simulink model "gm_DUALportRAMinterface_v3_vnl"  (R2024a)
settings: Solver=FixedStepDiscrete  StartTime=0.0  StopTime=0.1  RelTol=1e-3
undefined symbols (not defined in the file or in its folder): magnitude, Ts
libraries: hdlsllib x227, embmathops x6, simulink x2, hdlmdlgenlib x1, dsphdlxfrm2 x1
(part 1 of 6)
settings Model: Creator=Simon  LastModifiedBy=Simon
settings OptimizationCC: BlockReduction=off  ConditionallyExecuteInputs=off  DefaultParameterBehavior=Inlined  InheritOutputTypeSmallerThanSingle=on
settings DebuggingCC: AlgebraicLoopMsg=error  InheritedTsInSrcMsg=none  SingleTaskRateTransMsg=error  UnconnectedInputMsg=warning  UnconnectedOutputMsg=warning  UnconnectedLineMsg=warning
settings HardwareCC: ProdBitPerPointer=32  ProdBitPerSizeT=32  ProdBitPerPtrDiffT=32  ProdLargestAtomicFloat=None  ProdIntDivRoundTo=Undefined  ProdEndianess=Unspecified  ProdWordSize=32  ProdHWDeviceType=ASIC/FPGA->ASIC/FPGA  TargetBitPerPointer=64  TargetBitPerSizeT=64  TargetBitPerPtrDiffT=64  TargetLongLongMode=on  TargetIntDivRoundTo=Zero  TargetEndianess=LittleEndian  TargetWordSize=64  TargetHWDeviceType=Custom Processor->MATLAB Host Computer  ProdEqTarget=off

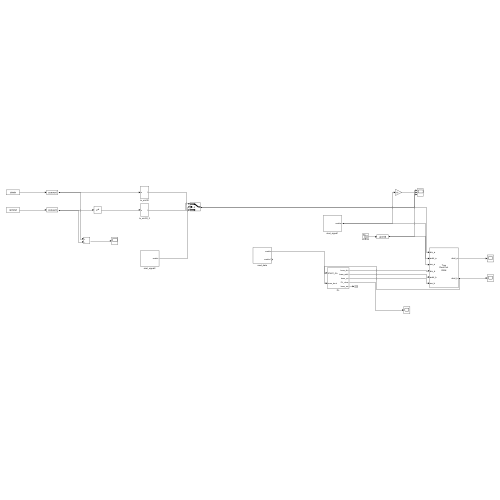
[thumbnail: Simulink's stored preview of the top-level diagram]
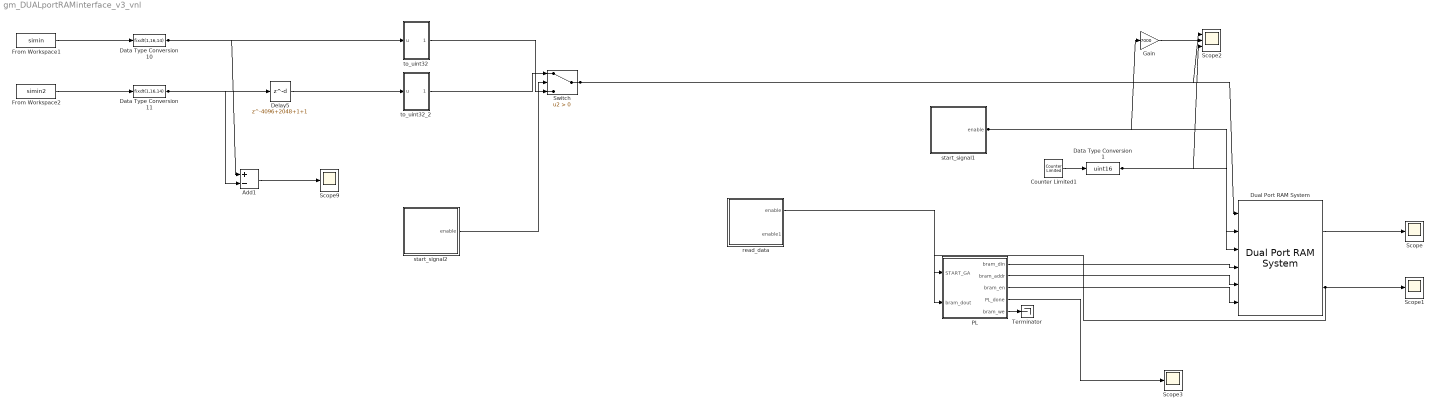
== system gm_DUALportRAMinterface_v3_vnl ==
  Add1 : Sum  Inputs=+-
  Counter Limited1 : simulink/Sources/Counter Limited  uplimit=14000  tsamp=Ts
  Data Type Conversion1 : DataTypeConversion  OutDataTypeStr=uint16  SaturateOnIntegerOverflow=off  RndMeth=Floor
  Data Type Conversion10 : DataTypeConversion  OutDataTypeStr=fixdt(1,16,14)  SaturateOnIntegerOverflow=off  RndMeth=Floor
  Data Type Conversion11 : DataTypeConversion  OutDataTypeStr=fixdt(1,16,14)  SaturateOnIntegerOverflow=off  RndMeth=Floor
  Delay5 : Delay  DelayLength=4096+2048+1+1  InitialCondition=0  SampleTime=Ts
  Dual Port RAM System : hdlsllib/HDL RAMs/Dual Port RAM System  RAMType=True dual port  AsyncRead=off  WriteOutputValue=New data  RAMInitialValue=0  allowBusInputs=off  WritesHaveOutput=on  NumReads=0  NumWrites=1  SimulateUsing=Code generation
  From Workspace1 : FromWorkspace  VariableName=simin  SampleTime=Ts
  From Workspace2 : FromWorkspace  VariableName=simin2  SampleTime=Ts
  Gain : Gain  Gain=7000
  PL : Subsystem
  Scope{,1,3,9} (4 alike) : Scope
  Scope2 : Scope  NumInputPorts=3
  Switch : Switch  Criteria=u2 > Threshold  SaturateOnIntegerOverflow=off  InputSameDT=off  OutDataTypeStr=Inherit: Same as first input
  Terminator : Terminator
  read_data : Subsystem
  start_signal1 : Subsystem
  start_signal2 : Subsystem
  to_uint32 : Subsystem
  to_uint32_2 : Subsystem
  wires:
  PL/5(bram_we) -> Terminator/1
  PL/4(PL_done) -> Scope3/1
  Data Type Conversion10/1 -> to_uint32/1(u), Add1/1
  Add1/1 -> Scope9/1
  Data Type Conversion11/1 -> Add1/2, Delay5/1
  Switch/1 -> Dual Port RAM System/1, Scope2/1
  Delay5/1 -> to_uint32_2/1(u)
  start_signal2/1(enable) -> Switch/2
  to_uint32_2/1(Out1) -> Switch/1
  to_uint32/1(Out1) -> Switch/3
  From Workspace2/1 -> Data Type Conversion11/1
  From Workspace1/1 -> Data Type Conversion10/1
  Dual Port RAM System/2 -> PL/2(bram_dout), Scope1/1
  read_data/1(enable) -> PL/1(START_GA)
  Gain/1 -> Scope2/2
  PL/3(bram_en) -> Dual Port RAM System/6
  PL/2(bram_addr) -> Dual Port RAM System/5
  PL/1(bram_din) -> Dual Port RAM System/4
  start_signal1/1(enable) -> Gain/1, Dual Port RAM System/3
  Data Type Conversion1/1 -> Dual Port RAM System/2, Scope2/3
  Counter Limited1/1 -> Data Type Conversion1/1
  Dual Port RAM System/1 -> Scope/1

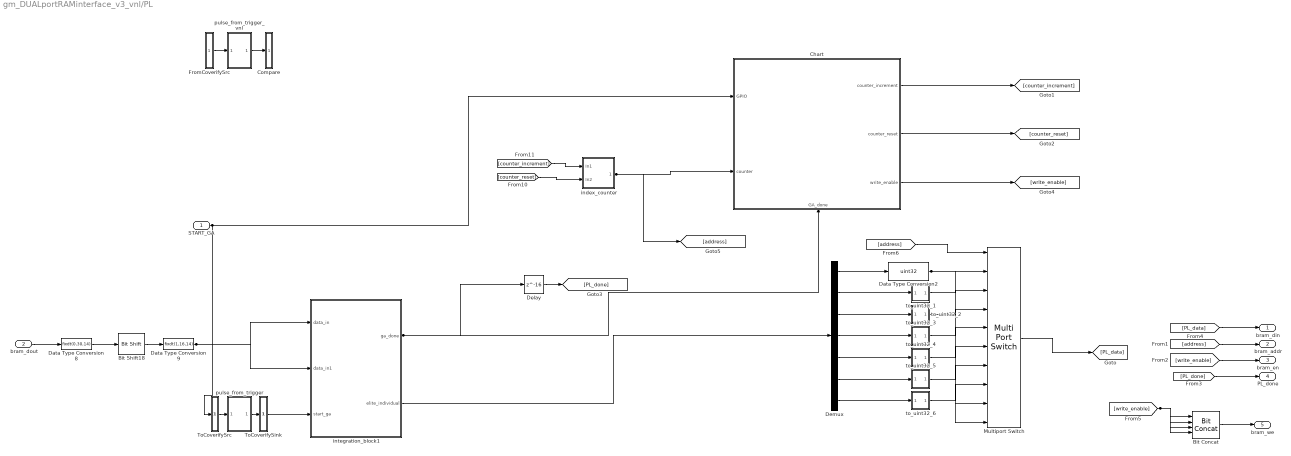
== system gm_DUALportRAMinterface_v3_vnl/PL ==
  START_GA : Inport
  bram_dout : Inport  Port=2
  Bit Concat : hdlsllib/Logic and Bit Operations/Bit Concat  numInputs=4
  Bit Shift18 : hdlsllib/Logic and Bit Operations/Bit Shift  mode=Shift Right Logical  N=14
  Chart : Stateflow chart  TreatAsAtomicUnit=on
      settings: PortSchema="{\"entries\":[{\"content\":{\"sides\":[{\"content\":{\"connectorIds\":[\"In2\",\"In3\"]},\"type\":\"ConnectorPlacement.EquallySpacedRectSide\",\"uuid\":\"f3ce331f-c708-4668-a9cb-fb327ea74ab5\"},{\"content\":{\"connectorIds\":[\"Out1\",\"Out2\",\"Out3\"],\"side\":\"RIGHT\"},\"type\":\"ConnectorPlacement.EquallySpacedRectSide\",\"uuid\":\"3766927a-abff-497d-9544-2098881ba174\"},{\"content\":{\"side\":\"TOP\"},\"type\":\"ConnectorPlacement.EquallySpacedRectSide\",\"uuid\":\"ebfe3d64-ee7d-4953-a6ba-e7e40988decf\"},{\"content\":{\"connectorIds\":[\"In1\"],\"side\":\"BOTTOM\"},\"type\":\"ConnectorPlacement.EquallySpacedRectSide\",\"uuid\":\"f39ceaf8-4df7-4e40-9de5-da7597831fb4\"}]},\"type\":\"ConnectorPlacement.EquallySpacedConnector\",\"uuid\":\"89f60450-5933-42bb-b72b-5f8ec55483e0\"}],\"packageUris\":[\"http://schema.mathworks.com/mf0/Connector/R2020b\"],\"version\":\"1.0\"}"
  Compare : Subsystem
      mask Display: disp('')
  Data Type Conversion2 : DataTypeConversion  OutDataTypeStr=uint32  SaturateOnIntegerOverflow=off  RndMeth=Floor
  Data Type Conversion8 : DataTypeConversion  OutDataTypeStr=fixdt(0,30,14)  SaturateOnIntegerOverflow=off  RndMeth=Floor
  Data Type Conversion9 : DataTypeConversion  OutDataTypeStr=fixdt(1,16,14)  SaturateOnIntegerOverflow=off  RndMeth=Floor
  Delay : Delay  DelayLength=16  InitialCondition=0  SampleTime=Ts
  Demux : Demux  Outputs=7
  FromCoverifySrc : Subsystem
      mask Display: disp('')
  Multiport Switch : MultiPortSwitch  DataPortOrder=Specify indices  Inputs=8  DataPortIndices={0,1,2,3,4,5,6,7}  DataPortForDefault=Additional data port  DiagnosticForDefault=None  SaturateOnIntegerOverflow=off  InputSameDT=off
  ToCoverifySink : Subsystem
      mask Display: disp('')
  ToCoverifySrc : Subsystem
      mask Display: disp('')
  index_counter : Subsystem
  integration_block1 : Subsystem
  pulse_from_trigger : Subsystem
  pulse_from_trigger_vnl : Subsystem
  to_uint32_1 : Subsystem
  to_uint32_2 : Subsystem
  to_uint32_3 : Subsystem
  to_uint32_4 : Subsystem
  to_uint32_5 : Subsystem
  to_uint32_6 : Subsystem
  bram_din : Outport
  bram_addr : Outport  Port=2
  bram_en : Outport  Port=3
  PL_done : Outport  Port=4
  bram_we : Outport  Port=5
  wires:
  Multiport Switch/1 -> [PL_data]
  [counter_reset] -> index_counter/2(In2)
  index_counter/1(index_counter) -> Chart/3(counter), [address]
  [address] -> bram_addr/1
  [counter_increment] -> index_counter/1(In1)
  [address] -> Multiport Switch/1
  Chart/3(write_enable) -> [write_enable]
  integration_block1/1(ga_done) -> Delay/1, Chart/1(GA_done)
  START_GA/1 -> Chart/2(GPIO), ToCoverifySrc/1(in1)
  Chart/2(counter_reset) -> [counter_reset]
  Chart/1(counter_increment) -> [counter_increment]
  [PL_data] -> bram_din/1
  [write_enable] -> bram_en/1
  integration_block1/2(elite_individual) -> Demux/1
  Demux/1 -> Data Type Conversion2/1
  Demux/2 -> to_uint32_1/1(u_port)
  Demux/3 -> to_uint32_2/1(u_port)
  Demux/4 -> to_uint32_3/1(u_port)
  Demux/5 -> to_uint32_4/1(u_port)
  Demux/6 -> to_uint32_5/1(u_port)
  Demux/7 -> to_uint32_6/1(u_port)
  Data Type Conversion2/1 -> Multiport Switch/10, Multiport Switch/9, Multiport Switch/2
  to_uint32_1/1(Out1) -> Multiport Switch/3
  to_uint32_2/1(Out1) -> Multiport Switch/4
  to_uint32_3/1(Out1) -> Multiport Switch/5
  to_uint32_4/1(Out1) -> Multiport Switch/6
  to_uint32_5/1(Out1) -> Multiport Switch/7
  to_uint32_6/1(Out1) -> Multiport Switch/8
  Data Type Conversion9/1 -> integration_block1/1(data_in), integration_block1/2(data_in1)
  Bit Shift18/1 -> Data Type Conversion9/1
  Data Type Conversion8/1 -> Bit Shift18/1
  bram_dout/1 -> Data Type Conversion8/1
  [PL_done] -> PL_done/1
  Delay/1 -> [PL_done]
  Bit Concat/1 -> bram_we/1
  [write_enable] -> Bit Concat/4, Bit Concat/3, Bit Concat/2, Bit Concat/1
  ToCoverifySrc/1(out1) -> pulse_from_trigger/1(In1)
  pulse_from_trigger/1(Out1) -> ToCoverifySink/1(in1)
  ToCoverifySink/1(out1) -> integration_block1/3(start_ga)
  FromCoverifySrc/1(out1) -> pulse_from_trigger_vnl/1(In1)
  pulse_from_trigger_vnl/1(Out1) -> Compare/1(in1)

== system gm_DUALportRAMinterface_v3_vnl/read_data ==
  Data Type Conversion1 : DataTypeConversion  Commented=on  OutDataTypeStr=boolean  SaturateOnIntegerOverflow=off  RndMeth=Floor
  Data Type Conversion29 : DataTypeConversion  OutDataTypeStr=boolean  SaturateOnIntegerOverflow=off  RndMeth=Floor
  Delay1 : Delay  Commented=on  DelayLength=1  InitialCondition=0  SampleTime=Ts
  Gain : Gain
  Gain1 : Gain  Commented=on
  Step1 : Step  Time=Ts*14000  SampleTime=Ts
  Step2 : Step  Commented=on  Time=Ts*14000  SampleTime=Ts
  XOR2 : Logic  Commented=on  Operator=XOR  IconShape=distinctive  AllPortsSameDT=off  OutDataTypeStr=boolean
  enable : Outport
  enable1 : Outport  Port=2
  wires:
  Gain1/1 -> Data Type Conversion1/1
  Step2/1 -> XOR2/1, Delay1/1
  Delay1/1 -> XOR2/2
  XOR2/1 -> Gain1/1
  Data Type Conversion1/1 -> enable1/1
  Data Type Conversion29/1 -> enable/1
  Gain/1 -> Data Type Conversion29/1
  Step1/1 -> Gain/1

== system gm_DUALportRAMinterface_v3_vnl/start_signal1 ==
  Data Type Conversion29 : DataTypeConversion  OutDataTypeStr=boolean  SaturateOnIntegerOverflow=off  RndMeth=Floor
  Delay2 : Delay  DelayLength=(4096+2048+1+1)*2  InitialCondition=0  SampleTime=Ts
  Gain : Gain
  Step1 : Step  Time=Ts*0  SampleTime=Ts
  XOR1 : Logic  Operator=XOR  IconShape=distinctive  AllPortsSameDT=off  OutDataTypeStr=boolean
  enable : Outport
  wires:
  XOR1/1 -> Gain/1
  Step1/1 -> Delay2/1, XOR1/1
  Delay2/1 -> XOR1/2
  Gain/1 -> Data Type Conversion29/1
  Data Type Conversion29/1 -> enable/1

== system gm_DUALportRAMinterface_v3_vnl/start_signal2 ==
  Data Type Conversion29 : DataTypeConversion  OutDataTypeStr=boolean  SaturateOnIntegerOverflow=off  RndMeth=Floor
  Delay2 : Delay  DelayLength=(4096+2048+1+1)*2  InitialCondition=0  SampleTime=Ts
  Gain : Gain
  Step1 : Step  Time=Ts*(4096+2048+1+1)  SampleTime=Ts
  XOR1 : Logic  Operator=XOR  IconShape=distinctive  AllPortsSameDT=off  OutDataTypeStr=boolean
  enable : Outport
  wires:
  Data Type Conversion29/1 -> enable/1
  Gain/1 -> Data Type Conversion29/1
  Delay2/1 -> XOR1/2
  Step1/1 -> XOR1/1, Delay2/1
  XOR1/1 -> Gain/1

== system gm_DUALportRAMinterface_v3_vnl/to_uint32 ==
  u : Inport
  Bit Concat2 : hdlsllib/Logic and Bit Operations/Bit Concat  numInputs=16
  Bit Shift19 : hdlsllib/Logic and Bit Operations/Bit Shift  mode=Shift Left Logical  N=1
  Bit Shift20 : hdlsllib/Logic and Bit Operations/Bit Shift  mode=Shift Left Logical  N=10
  Bit Shift21 : hdlsllib/Logic and Bit Operations/Bit Shift  mode=Shift Right Logical  N=1
  Bit Shift22 : hdlsllib/Logic and Bit Operations/Bit Shift  mode=Shift Left Logical  N=11
  Bit Shift23 : hdlsllib/Logic and Bit Operations/Bit Shift  mode=Shift Left Logical  N=12
  Bit Shift24 : hdlsllib/Logic and Bit Operations/Bit Shift  mode=Shift Left Logical  N=13
  Bit Shift25 : hdlsllib/Logic and Bit Operations/Bit Shift  mode=Shift Left Logical  N=14
  Bit Shift26 : hdlsllib/Logic and Bit Operations/Bit Shift  mode=Shift Left Logical  N=2
  Bit Shift27 : hdlsllib/Logic and Bit Operations/Bit Shift  mode=Shift Left Logical  N=3
  Bit Shift28 : hdlsllib/Logic and Bit Operations/Bit Shift  mode=Shift Left Logical  N=4
  Bit Shift29 : hdlsllib/Logic and Bit Operations/Bit Shift  mode=Shift Left Logical  N=5
  Bit Shift30 : hdlsllib/Logic and Bit Operations/Bit Shift  mode=Shift Left Logical  N=6
  Bit Shift31 : hdlsllib/Logic and Bit Operations/Bit Shift  mode=Shift Left Logical  N=7
  Bit Shift32 : hdlsllib/Logic and Bit Operations/Bit Shift  mode=Shift Left Logical  N=8
  Bit Shift33 : hdlsllib/Logic and Bit Operations/Bit Shift  mode=Shift Left Logical  N=9
  Data Type Conversion{12..16,26,34..43} (16 alike) : DataTypeConversion  OutDataTypeStr=fixdt(0,1,0)  SaturateOnIntegerOverflow=off  RndMeth=Floor
  Data Type Conversion44 : DataTypeConversion  OutDataTypeStr=uint32  SaturateOnIntegerOverflow=off  RndMeth=Floor
  Out1 : Outport
  wires:
  Data Type Conversion14/1 -> Bit Concat2/10
  Bit Concat2/1 -> Data Type Conversion44/1
  Bit Shift26/1 -> Data Type Conversion35/1
  Bit Shift21/1 -> Data Type Conversion13/1
  Bit Shift28/1 -> Data Type Conversion26/1
  Data Type Conversion37/1 -> Bit Concat2/16
  Bit Shift29/1 -> Data Type Conversion16/1
  Bit Shift23/1 -> Data Type Conversion39/1
  Data Type Conversion41/1 -> Bit Concat2/12
  Bit Shift24/1 -> Data Type Conversion38/1
  Bit Shift33/1 -> Data Type Conversion42/1
  Data Type Conversion16/1 -> Bit Concat2/7
  Data Type Conversion43/1 -> Bit Concat2/9
  Data Type Conversion34/1 -> Bit Concat2/5
  Data Type Conversion39/1 -> Bit Concat2/14
  Bit Shift32/1 -> Data Type Conversion14/1
  Data Type Conversion12/1 -> Bit Concat2/2
  Bit Shift30/1 -> Data Type Conversion15/1
  Data Type Conversion15/1 -> Bit Concat2/8
  Bit Shift25/1 -> Data Type Conversion37/1
  Data Type Conversion38/1 -> Bit Concat2/15
  Bit Shift19/1 -> Data Type Conversion36/1
  Data Type Conversion42/1 -> Bit Concat2/11
  Data Type Conversion35/1 -> Bit Concat2/4
  Data Type Conversion44/1 -> Out1/1
  Data Type Conversion26/1 -> Bit Concat2/6
  Bit Shift31/1 -> Data Type Conversion43/1
  Data Type Conversion40/1 -> Bit Concat2/13
  Data Type Conversion13/1 -> Bit Concat2/1
  Bit Shift20/1 -> Data Type Conversion41/1
  u/1 -> Bit Shift25/1, Bit Shift24/1, Bit Shift23/1, Bit Shift22/1, Bit Shift20/1, Bit Shift33/1, Bit Shift32/1, Bit Shift31/1, Bit Shift30/1, Bit Shift29/1, Bit Shift28/1, Bit Shift27/1, Bit Shift26/1, Bit Shift19/1, Data Type Conversion12/1, Bit Shift21/1
  Data Type Conversion36/1 -> Bit Concat2/3
  Bit Shift27/1 -> Data Type Conversion34/1
  Bit Shift22/1 -> Data Type Conversion40/1

== system gm_DUALportRAMinterface_v3_vnl/to_uint32_2 ==
  u : Inport
  Bit Concat2 : hdlsllib/Logic and Bit Operations/Bit Concat  numInputs=16
  Bit Shift19 : hdlsllib/Logic and Bit Operations/Bit Shift  mode=Shift Left Logical  N=1
  Bit Shift20 : hdlsllib/Logic and Bit Operations/Bit Shift  mode=Shift Left Logical  N=10
  Bit Shift21 : hdlsllib/Logic and Bit Operations/Bit Shift  mode=Shift Right Logical  N=1
  Bit Shift22 : hdlsllib/Logic and Bit Operations/Bit Shift  mode=Shift Left Logical  N=11
  Bit Shift23 : hdlsllib/Logic and Bit Operations/Bit Shift  mode=Shift Left Logical  N=12
  Bit Shift24 : hdlsllib/Logic and Bit Operations/Bit Shift  mode=Shift Left Logical  N=13
  Bit Shift25 : hdlsllib/Logic and Bit Operations/Bit Shift  mode=Shift Left Logical  N=14
  Bit Shift26 : hdlsllib/Logic and Bit Operations/Bit Shift  mode=Shift Left Logical  N=2
  Bit Shift27 : hdlsllib/Logic and Bit Operations/Bit Shift  mode=Shift Left Logical  N=3
  Bit Shift28 : hdlsllib/Logic and Bit Operations/Bit Shift  mode=Shift Left Logical  N=4
  Bit Shift29 : hdlsllib/Logic and Bit Operations/Bit Shift  mode=Shift Left Logical  N=5
  Bit Shift30 : hdlsllib/Logic and Bit Operations/Bit Shift  mode=Shift Left Logical  N=6
  Bit Shift31 : hdlsllib/Logic and Bit Operations/Bit Shift  mode=Shift Left Logical  N=7
  Bit Shift32 : hdlsllib/Logic and Bit Operations/Bit Shift  mode=Shift Left Logical  N=8
  Bit Shift33 : hdlsllib/Logic and Bit Operations/Bit Shift  mode=Shift Left Logical  N=9
  Data Type Conversion{12..16,26,34..43} (16 alike) : DataTypeConversion  OutDataTypeStr=fixdt(0,1,0)  SaturateOnIntegerOverflow=off  RndMeth=Floor
  Data Type Conversion44 : DataTypeConversion  OutDataTypeStr=uint32  SaturateOnIntegerOverflow=off  RndMeth=Floor
  Out1 : Outport
  wires:
  Bit Shift22/1 -> Data Type Conversion40/1
  Bit Shift27/1 -> Data Type Conversion34/1
  Data Type Conversion36/1 -> Bit Concat2/3
  u/1 -> Bit Shift21/1, Data Type Conversion12/1, Bit Shift19/1, Bit Shift26/1, Bit Shift27/1, Bit Shift28/1, Bit Shift29/1, Bit Shift30/1, Bit Shift31/1, Bit Shift32/1, Bit Shift33/1, Bit Shift20/1, Bit Shift22/1, Bit Shift23/1, Bit Shift24/1, Bit Shift25/1
  Bit Shift20/1 -> Data Type Conversion41/1
  Data Type Conversion13/1 -> Bit Concat2/1
  Data Type Conversion40/1 -> Bit Concat2/13
  Bit Shift31/1 -> Data Type Conversion43/1
  Data Type Conversion26/1 -> Bit Concat2/6
  Data Type Conversion44/1 -> Out1/1
  Data Type Conversion35/1 -> Bit Concat2/4
  Data Type Conversion42/1 -> Bit Concat2/11
  Bit Shift19/1 -> Data Type Conversion36/1
  Data Type Conversion38/1 -> Bit Concat2/15
  Bit Shift25/1 -> Data Type Conversion37/1
  Data Type Conversion15/1 -> Bit Concat2/8
  Bit Shift30/1 -> Data Type Conversion15/1
  Data Type Conversion12/1 -> Bit Concat2/2
  Bit Shift32/1 -> Data Type Conversion14/1
  Data Type Conversion39/1 -> Bit Concat2/14
  Data Type Conversion34/1 -> Bit Concat2/5
  Data Type Conversion43/1 -> Bit Concat2/9
  Data Type Conversion16/1 -> Bit Concat2/7
  Bit Shift33/1 -> Data Type Conversion42/1
  Bit Shift24/1 -> Data Type Conversion38/1
  Data Type Conversion41/1 -> Bit Concat2/12
  Bit Shift23/1 -> Data Type Conversion39/1
  Bit Shift29/1 -> Data Type Conversion16/1
  Data Type Conversion37/1 -> Bit Concat2/16
  Bit Shift28/1 -> Data Type Conversion26/1
  Bit Shift21/1 -> Data Type Conversion13/1
  Bit Shift26/1 -> Data Type Conversion35/1
  Bit Concat2/1 -> Data Type Conversion44/1
  Data Type Conversion14/1 -> Bit Concat2/10

== system gm_DUALportRAMinterface_v3_vnl/PL/Compare ==
  in1 : Inport
  Assert_Out1 : Subsystem
      settings: LibrarySourceBlock=hdlmdlgenlib/AssertEq
  CleanupScopes : Subsystem
      settings: OpenFcn=|
      | blkName = gcb; %self block
      | idx = regexp(blkName, '/CleanupScopes$', 'once');
      | blkParent = blkName(1:idx-1);
      | blks=find_system(blkParent, 'LookUnderMasks', 'all','blocktype', 'Scope');
      | for itr = 1:length(blks)
      | 	 hScopeCfg = get_param(blks{itr},'ScopeConfiguration');
      | 	 hScopeCfg.Visible = ~ hScopeCfg.Visible;
      | end
      | drawnow;
      mask Display: fprintf(message('hdlcoder:cosim:vnl_dblclick').getString());
  Enable : Subsystem
      settings: OpenFcn=|
      | blkName = gcb;
      | idx = regexp(blkName, '/Enable$', 'once');
      | blkParent = blkName(1:idx-1);
      | blks=find_system(blkParent, 'LookUnderMasks', 'all','blocktype', 'Assertion');
      | e = get_param(blks{1}, 'Enabled');
      | if strcmp(e, 'on'), f= 'off';, else, f = 'on';, end
      | for ii=1:length(blks), set_param(blks{ii}, 'Enabled', f);, end
      | set_param(gcb, 'MaskDisplay',['fprintf(message(''hdlcoder:cosim:vnl_dblclick_assertions'',','''',upper(e),'''',').getString())']);
      mask Display: fprintf(message('hdlcoder:cosim:vnl_dblclick_assertions','OFF').getString());
  wires:
  in1/1 -> Assert_Out1/1(cosim)
  [out1] -> Assert_Out1/2(dut)

== system gm_DUALportRAMinterface_v3_vnl/PL/FromCoverifySrc ==
  out1 : Outport
  wires:
  [in1] -> out1/1

== system gm_DUALportRAMinterface_v3_vnl/PL/ToCoverifySink ==
  in1 : Inport
  out1 : Outport
  tag scope: out1=global
  wires:
  in1/1 -> out1/1, [out1]

== system gm_DUALportRAMinterface_v3_vnl/PL/ToCoverifySrc ==
  in1 : Inport
  out1 : Outport
  tag scope: in1=global
  wires:
  in1/1 -> out1/1, [in1]

== system gm_DUALportRAMinterface_v3_vnl/PL/index_counter ==
  In1 : Inport
  In2 : Inport  Port=2
  Add : Sum  OutDataTypeStr=Inherit: Same as first input
  Constant18 : Constant  OutDataTypeStr=fixdt(0,16,0)  SampleTime=Ts
  Constant19 : Constant  Value=0  OutDataTypeStr=fixdt(0,16,0)  SampleTime=Ts
  Constant20 : Constant  Value=0  OutDataTypeStr=uint16  SampleTime=Ts
  Delay : Delay  DelayLength=1  InitialCondition=0  SampleTime=Ts
  Switch : Switch  Criteria=u2 > Threshold  SaturateOnIntegerOverflow=off  InputSameDT=off  OutDataTypeStr=Inherit: Same as first input
  Switch8 : Switch  Criteria=u2 > Threshold  SaturateOnIntegerOverflow=off  InputSameDT=off  OutDataTypeStr=Inherit: Same as first input
  index_counter : Outport
  wires:
  In1/1 -> Switch/2
  Constant18/1 -> Switch/1
  Constant20/1 -> Switch8/1
  Add/1 -> Delay/1
  In2/1 -> Switch8/2
  Delay/1 -> Switch8/3, index_counter/1
  Switch/1 -> Add/1
  Switch8/1 -> Add/2
  Constant19/1 -> Switch/3

== system gm_DUALportRAMinterface_v3_vnl/PL/integration_block1 ==
  data_in : Inport
  data_in1 : Inport  Port=2
  start_ga : Inport  Port=3
  D2 : Subsystem
      settings: PortSchema="{\"entries\":[{\"content\":{\"sides\":[{\"content\":{\"connectorIds\":[\"In1\",\"In2\"]},\"type\":\"ConnectorPlacement.EquallySpacedRectSide\",\"uuid\":\"5abe48ab-1b34-4cb0-8d41-07cb17904e64\"},{\"content\":{\"connectorIds\":[\"Out1\"],\"side\":\"RIGHT\"},\"type\":\"ConnectorPlacement.EquallySpacedRectSide\",\"uuid\":\"19bc24ff-88f3-42df-af8e-ecb9c1c6119c\"},{\"content\":{\"connectorIds\":[\"In3\"],\"side\":\"TOP\"},\"type\":\"ConnectorPlacement.EquallySpacedRectSide\",\"uuid\":\"46fc65c4-6cee-4e0a-9107-9d106d0a52a5\"},{\"content\":{\"connectorIds\":[\"In4\"],\"side\":\"BOTTOM\"},\"type\":\"ConnectorPlacement.EquallySpacedRectSide\",\"uuid\":\"10a5fc09-3948-4556-8b0c-050853396926\"}]},\"type\":\"ConnectorPlacement.EquallySpacedConnector\",\"uuid\":\"9cc35bfe-5b00-42b0-9811-425d4f0f8f7b\"}],\"packageUris\":[\"http://schema.mathworks.com/mf0/Connector/R2020b\"],\"version\":\"1.0\"}"
  Delay : Delay  DelayLength=6145  InitialCondition=0  UseCircularBuffer=on  SampleTime=Ts
  Delay3 : Delay  DelayLength=1  InitialCondition=0  SampleTime=Ts
  FFT : dsphdlxfrm2/FFT  Architecture=Burst Radix 2  FFTLengthSource=Property  FFTLength=4096  FFTLengthMax=1024  ComplexMultiplication=Use 4 multipliers and 2 adders  BitReversedOutput=off  BitReversedInput=off  Normalize=off  SimulateUsing=Code generation  RoundingMethod=Floor  ResetInputPort=on  StartOutputPort=off  EndOutputPort=off
  FIFO_system1 : Subsystem
  FIFO_system3 : Subsystem
  GA_main : Subsystem
      settings: PortSchema="{\"entries\":[{\"content\":{\"sides\":[{\"content\":{\"connectorIds\":[\"In1\",\"In2\",\"In3\",\"In4\",\"In5\",\"In6\",\"In7\",\"In8\",\"In9\",\"In10\",\"In11\"]},\"type\":\"ConnectorPlacement.EquallySpacedRectSide\",\"uuid\":\"daccc056-a93f-45e5-9369-71b73e32651e\"},{\"content\":{\"connectorIds\":[\"Out1\",\"Out2\"],\"side\":\"RIGHT\"},\"type\":\"ConnectorPlacement.EquallySpacedRectSide\",\"uuid\":\"82109161-9ebe-455f-914b-56f9927b10eb\"},{\"content\":{\"connectorIds\":[\"Out3\",\"Out4\",\"Out5\",\"In12\",\"In13\"],\"side\":\"TOP\"},\"type\":\"ConnectorPlacement.EquallySpacedRectSide\",\"uuid\":\"07b2e20b-bb92-4769-b746-3d44a115cdd8\"}]},\"type\":\"ConnectorPlacement.EquallySpacedConnector\",\"uuid\":\"c9f522d4-4f80-4900-b8a5-3110692e6ae8\"}],\"packageUris\":[\"http://schema.mathworks.com/mf0/Connector/R2020b\"],\"version\":\"1.0\"}"
  Subsystem : Subsystem
  Sum : Sum  Inputs=|+-  OutDataTypeStr=Inherit: Same as first input
  Terminator : Terminator
  Terminator1 : Terminator
  Terminator2 : Terminator
  accumulator_scorer : Subsystem
  ga_done : Outport
  elite_individual : Outport  Port=2
  wires:
  GA_main/1(elite_individual) -> elite_individual/1
  FIFO_system1/4(FIFO_full) -> FIFO_system3/3(load_fifo)
  Subsystem/9(random_sample_out) -> GA_main/11(tb_random_sample)
  Subsystem/8(a4_random_out) -> GA_main/10(a4rnd)
  Subsystem/7(a3_random_out) -> GA_main/9(a3rnd)
  Subsystem/6(a2_random_out) -> GA_main/8(a2rnd)
  Subsystem/5(b4_random_out) -> GA_main/7(b4rnd)
  Subsystem/4(b3_random_out) -> GA_main/6(b3rnd)
  Subsystem/3(b2_random_out) -> GA_main/5(b2rnd)
  Subsystem/2(random_method_out) -> GA_main/4(random_method)
  Subsystem/1(random_gene_out) -> GA_main/3(random_gene)
  Delay/1 -> D2/3(reset_D2)
  Sum/1 -> FFT/1
  FIFO_system3/4(FIFO_full) -> GA_main/12(FIFO_full)
  FIFO_system1/3(reset_fft) -> FFT/3, Delay/1
  FIFO_system1/2(data_valid) -> FFT/2
  data_in1/1 -> FIFO_system3/1(data_in)
  Delay3/1 -> GA_main/13(score_done)
  FIFO_system3/3(reset_fft) -> Terminator2/1
  accumulator_scorer/2(individual_score_valid) -> Delay3/1
  GA_main/3(individual_to_d2) -> D2/4(Individual_input)
  FIFO_system3/1(data_out) -> D2/1(GAerror)
  GA_main/2(ga_done) -> ga_done/1
  data_in/1 -> FIFO_system1/1(data_in)
  GA_main/4(FIFO_out_en) -> FIFO_system1/2(enable_output), FIFO_system3/2(enable_output), D2/2(push_individual)
  GA_main/5(load_fifo) -> FIFO_system1/3(load_fifo)
  FFT/3 -> Terminator/1
  FFT/1 -> accumulator_scorer/1(data_in)
  D2/1(response) -> Sum/2
  start_ga/1 -> Subsystem/1(enable), GA_main/1(start_ga)
  FIFO_system1/1(data_out) -> Sum/1
  accumulator_scorer/1(individual_score) -> GA_main/2(score_result)
  FIFO_system3/2(data_valid) -> Terminator1/1
  FFT/2 -> accumulator_scorer/2(valid_fft)

== system gm_DUALportRAMinterface_v3_vnl/PL/pulse_from_trigger ==
  In1 : Inport
  Delay1 : Delay  DelayLength=1  InitialCondition=0  SampleTime=Ts
  Logical Operator : Logic  IconShape=distinctive  AllPortsSameDT=off  OutDataTypeStr=boolean
  Logical Operator1 : Logic  Operator=XOR  IconShape=distinctive  AllPortsSameDT=off  OutDataTypeStr=boolean
  Out1 : Outport
  wires:
  In1/1 -> Logical Operator1/1, Logical Operator/1, Delay1/1
  Delay1/1 -> Logical Operator/2
  Logical Operator/1 -> Logical Operator1/2
  Logical Operator1/1 -> Out1/1

== system gm_DUALportRAMinterface_v3_vnl/PL/pulse_from_trigger_vnl ==
  In1 : Inport
  Delay1 : Delay  DelayLength=1  InitialCondition=0  SampleTime=Ts
  Logical Operator : Logic  IconShape=distinctive  AllPortsSameDT=off  OutDataTypeStr=boolean
  Logical Operator1 : Logic  Operator=XOR  IconShape=distinctive  AllPortsSameDT=off  OutDataTypeStr=boolean
  Out1 : Outport
  wires:
  Logical Operator1/1 -> Out1/1
  Logical Operator/1 -> Logical Operator1/2
  Delay1/1 -> Logical Operator/2
  In1/1 -> Delay1/1, Logical Operator/1, Logical Operator1/1

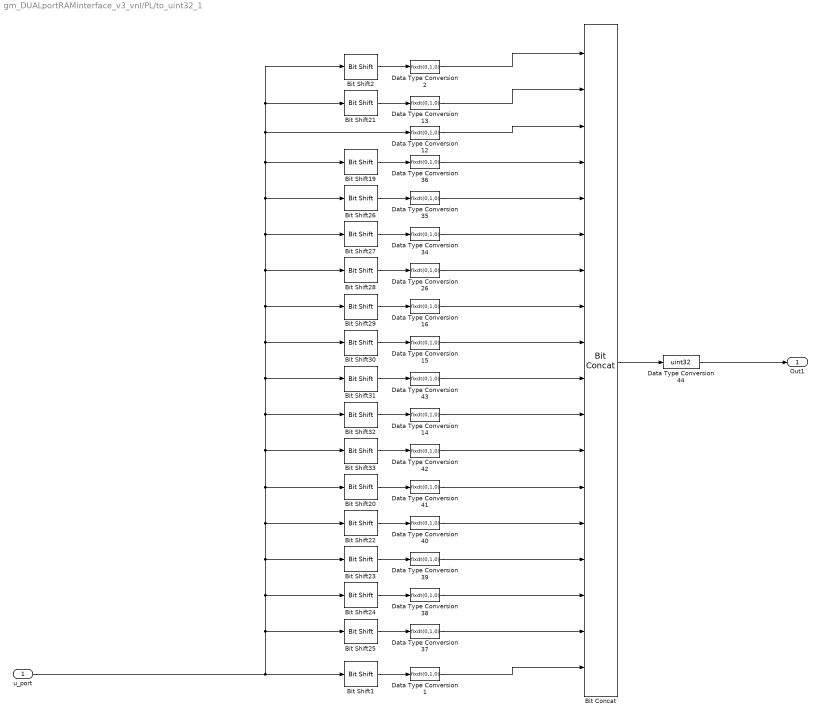
== system gm_DUALportRAMinterface_v3_vnl/PL/to_uint32_1 ==
  u_port : Inport
  Bit Concat : hdlsllib/Logic and Bit Operations/Bit Concat  numInputs=18
  Bit Shift1 : hdlsllib/Logic and Bit Operations/Bit Shift  mode=Shift Left Logical  N=15
  Bit Shift19 : hdlsllib/Logic and Bit Operations/Bit Shift  mode=Shift Left Logical  N=1
  Bit Shift2 : hdlsllib/Logic and Bit Operations/Bit Shift  mode=Shift Right Logical  N=16
  Bit Shift20 : hdlsllib/Logic and Bit Operations/Bit Shift  mode=Shift Left Logical  N=10
  Bit Shift21 : hdlsllib/Logic and Bit Operations/Bit Shift  mode=Shift Right Logical  N=1
  Bit Shift22 : hdlsllib/Logic and Bit Operations/Bit Shift  mode=Shift Left Logical  N=11
  Bit Shift23 : hdlsllib/Logic and Bit Operations/Bit Shift  mode=Shift Left Logical  N=12
  Bit Shift24 : hdlsllib/Logic and Bit Operations/Bit Shift  mode=Shift Left Logical  N=13
  Bit Shift25 : hdlsllib/Logic and Bit Operations/Bit Shift  mode=Shift Left Logical  N=14
  Bit Shift26 : hdlsllib/Logic and Bit Operations/Bit Shift  mode=Shift Left Logical  N=2
  Bit Shift27 : hdlsllib/Logic and Bit Operations/Bit Shift  mode=Shift Left Logical  N=3
  Bit Shift28 : hdlsllib/Logic and Bit Operations/Bit Shift  mode=Shift Left Logical  N=4
  Bit Shift29 : hdlsllib/Logic and Bit Operations/Bit Shift  mode=Shift Left Logical  N=5
  Bit Shift30 : hdlsllib/Logic and Bit Operations/Bit Shift  mode=Shift Left Logical  N=6
  Bit Shift31 : hdlsllib/Logic and Bit Operations/Bit Shift  mode=Shift Left Logical  N=7
  Bit Shift32 : hdlsllib/Logic and Bit Operations/Bit Shift  mode=Shift Left Logical  N=8
  Bit Shift33 : hdlsllib/Logic and Bit Operations/Bit Shift  mode=Shift Left Logical  N=9
  Data Type Conversion{1..2,12..16,26,34..43} (18 alike) : DataTypeConversion  OutDataTypeStr=fixdt(0,1,0)  SaturateOnIntegerOverflow=off  RndMeth=Floor
  Data Type Conversion44 : DataTypeConversion  OutDataTypeStr=uint32  SaturateOnIntegerOverflow=off  RndMeth=Floor
  Out1 : Outport
  wires:
  Bit Concat/1 -> Data Type Conversion44/1
  u_port/1 -> Bit Shift1/1, Bit Shift21/1, Bit Shift2/1, Data Type Conversion12/1, Bit Shift19/1, Bit Shift26/1, Bit Shift27/1, Bit Shift28/1, Bit Shift29/1, Bit Shift30/1, Bit Shift31/1, Bit Shift32/1, Bit Shift33/1, Bit Shift20/1, Bit Shift22/1, Bit Shift23/1, Bit Shift24/1, Bit Shift25/1
  Data Type Conversion14/1 -> Bit Concat/11
  Data Type Conversion1/1 -> Bit Concat/18
  Data Type Conversion2/1 -> Bit Concat/1
  Data Type Conversion26/1 -> Bit Concat/7
  Bit Shift21/1 -> Data Type Conversion13/1
  Data Type Conversion12/1 -> Bit Concat/3
  Bit Shift27/1 -> Data Type Conversion34/1
  Bit Shift22/1 -> Data Type Conversion40/1
  Bit Shift20/1 -> Data Type Conversion41/1
  Bit Shift31/1 -> Data Type Conversion43/1
  Data Type Conversion39/1 -> Bit Concat/15
  Data Type Conversion15/1 -> Bit Concat/9
  Data Type Conversion43/1 -> Bit Concat/10
  Bit Shift33/1 -> Data Type Conversion42/1
  Bit Shift23/1 -> Data Type Conversion39/1
  Bit Shift25/1 -> Data Type Conversion37/1
  Data Type Conversion41/1 -> Bit Concat/13
  Bit Shift2/1 -> Data Type Conversion2/1
  Bit Shift29/1 -> Data Type Conversion16/1
  Bit Shift26/1 -> Data Type Conversion35/1
  Data Type Conversion34/1 -> Bit Concat/6
  Bit Shift28/1 -> Data Type Conversion26/1
  Data Type Conversion36/1 -> Bit Concat/4
  Bit Shift24/1 -> Data Type Conversion38/1
  Bit Shift1/1 -> Data Type Conversion1/1
  Data Type Conversion35/1 -> Bit Concat/5
  Data Type Conversion16/1 -> Bit Concat/8
  Bit Shift19/1 -> Data Type Conversion36/1
  Data Type Conversion13/1 -> Bit Concat/2
  Bit Shift30/1 -> Data Type Conversion15/1
  Data Type Conversion38/1 -> Bit Concat/16
  Data Type Conversion37/1 -> Bit Concat/17
  Data Type Conversion40/1 -> Bit Concat/14
  Bit Shift32/1 -> Data Type Conversion14/1
  Data Type Conversion42/1 -> Bit Concat/12
  Data Type Conversion44/1 -> Out1/1

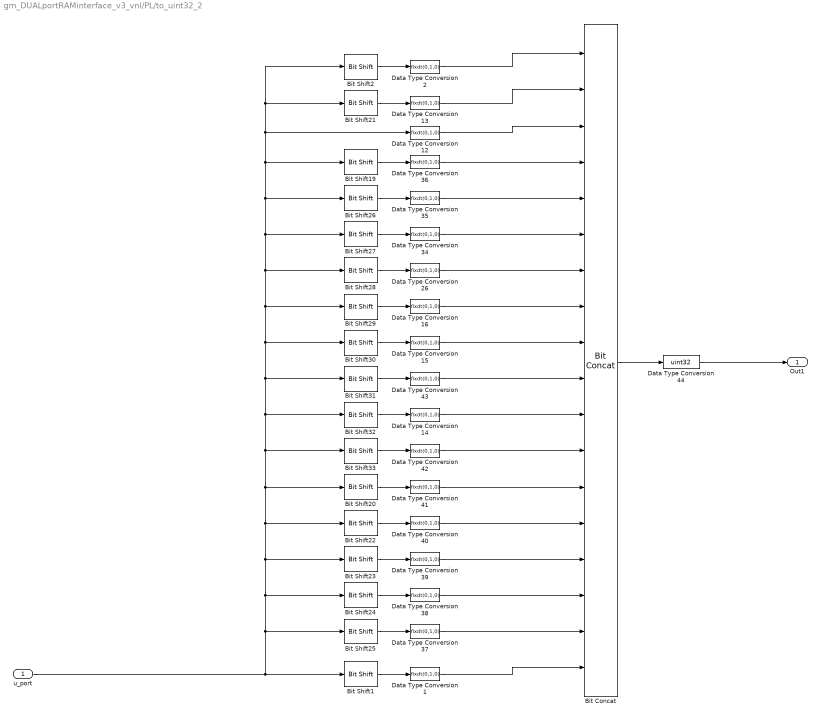
== system gm_DUALportRAMinterface_v3_vnl/PL/to_uint32_2 ==
  u_port : Inport
  Bit Concat : hdlsllib/Logic and Bit Operations/Bit Concat  numInputs=18
  Bit Shift1 : hdlsllib/Logic and Bit Operations/Bit Shift  mode=Shift Left Logical  N=15
  Bit Shift19 : hdlsllib/Logic and Bit Operations/Bit Shift  mode=Shift Left Logical  N=1
  Bit Shift2 : hdlsllib/Logic and Bit Operations/Bit Shift  mode=Shift Right Logical  N=16
  Bit Shift20 : hdlsllib/Logic and Bit Operations/Bit Shift  mode=Shift Left Logical  N=10
  Bit Shift21 : hdlsllib/Logic and Bit Operations/Bit Shift  mode=Shift Right Logical  N=1
  Bit Shift22 : hdlsllib/Logic and Bit Operations/Bit Shift  mode=Shift Left Logical  N=11
  Bit Shift23 : hdlsllib/Logic and Bit Operations/Bit Shift  mode=Shift Left Logical  N=12
  Bit Shift24 : hdlsllib/Logic and Bit Operations/Bit Shift  mode=Shift Left Logical  N=13
  Bit Shift25 : hdlsllib/Logic and Bit Operations/Bit Shift  mode=Shift Left Logical  N=14
  Bit Shift26 : hdlsllib/Logic and Bit Operations/Bit Shift  mode=Shift Left Logical  N=2
  Bit Shift27 : hdlsllib/Logic and Bit Operations/Bit Shift  mode=Shift Left Logical  N=3
  Bit Shift28 : hdlsllib/Logic and Bit Operations/Bit Shift  mode=Shift Left Logical  N=4
  Bit Shift29 : hdlsllib/Logic and Bit Operations/Bit Shift  mode=Shift Left Logical  N=5
  Bit Shift30 : hdlsllib/Logic and Bit Operations/Bit Shift  mode=Shift Left Logical  N=6
  Bit Shift31 : hdlsllib/Logic and Bit Operations/Bit Shift  mode=Shift Left Logical  N=7
  Bit Shift32 : hdlsllib/Logic and Bit Operations/Bit Shift  mode=Shift Left Logical  N=8
  Bit Shift33 : hdlsllib/Logic and Bit Operations/Bit Shift  mode=Shift Left Logical  N=9
  Data Type Conversion{1..2,12..16,26,34..43} (18 alike) : DataTypeConversion  OutDataTypeStr=fixdt(0,1,0)  SaturateOnIntegerOverflow=off  RndMeth=Floor
  Data Type Conversion44 : DataTypeConversion  OutDataTypeStr=uint32  SaturateOnIntegerOverflow=off  RndMeth=Floor
  Out1 : Outport
  wires:
  Data Type Conversion44/1 -> Out1/1
  Data Type Conversion42/1 -> Bit Concat/12
  Bit Shift32/1 -> Data Type Conversion14/1
  Data Type Conversion40/1 -> Bit Concat/14
  Data Type Conversion37/1 -> Bit Concat/17
  Data Type Conversion38/1 -> Bit Concat/16
  Bit Shift30/1 -> Data Type Conversion15/1
  Data Type Conversion13/1 -> Bit Concat/2
  Bit Shift19/1 -> Data Type Conversion36/1
  Data Type Conversion16/1 -> Bit Concat/8
  Data Type Conversion35/1 -> Bit Concat/5
  Bit Shift1/1 -> Data Type Conversion1/1
  Bit Shift24/1 -> Data Type Conversion38/1
  Data Type Conversion36/1 -> Bit Concat/4
  Bit Shift28/1 -> Data Type Conversion26/1
  Data Type Conversion34/1 -> Bit Concat/6
  Bit Shift26/1 -> Data Type Conversion35/1
  Bit Shift29/1 -> Data Type Conversion16/1
  Bit Shift2/1 -> Data Type Conversion2/1
  Data Type Conversion41/1 -> Bit Concat/13
  Bit Shift25/1 -> Data Type Conversion37/1
  Bit Shift23/1 -> Data Type Conversion39/1
  Bit Shift33/1 -> Data Type Conversion42/1
  Data Type Conversion43/1 -> Bit Concat/10
  Data Type Conversion15/1 -> Bit Concat/9
  Data Type Conversion39/1 -> Bit Concat/15
  Bit Shift31/1 -> Data Type Conversion43/1
  Bit Shift20/1 -> Data Type Conversion41/1
  Bit Shift22/1 -> Data Type Conversion40/1
  Bit Shift27/1 -> Data Type Conversion34/1
  Data Type Conversion12/1 -> Bit Concat/3
  Bit Shift21/1 -> Data Type Conversion13/1
  Data Type Conversion26/1 -> Bit Concat/7
  Data Type Conversion2/1 -> Bit Concat/1
  Data Type Conversion1/1 -> Bit Concat/18
  Data Type Conversion14/1 -> Bit Concat/11
  u_port/1 -> Bit Shift25/1, Bit Shift24/1, Bit Shift23/1, Bit Shift22/1, Bit Shift20/1, Bit Shift33/1, Bit Shift32/1, Bit Shift31/1, Bit Shift30/1, Bit Shift29/1, Bit Shift28/1, Bit Shift27/1, Bit Shift26/1, Bit Shift19/1, Data Type Conversion12/1, Bit Shift2/1, Bit Shift21/1, Bit Shift1/1
  Bit Concat/1 -> Data Type Conversion44/1

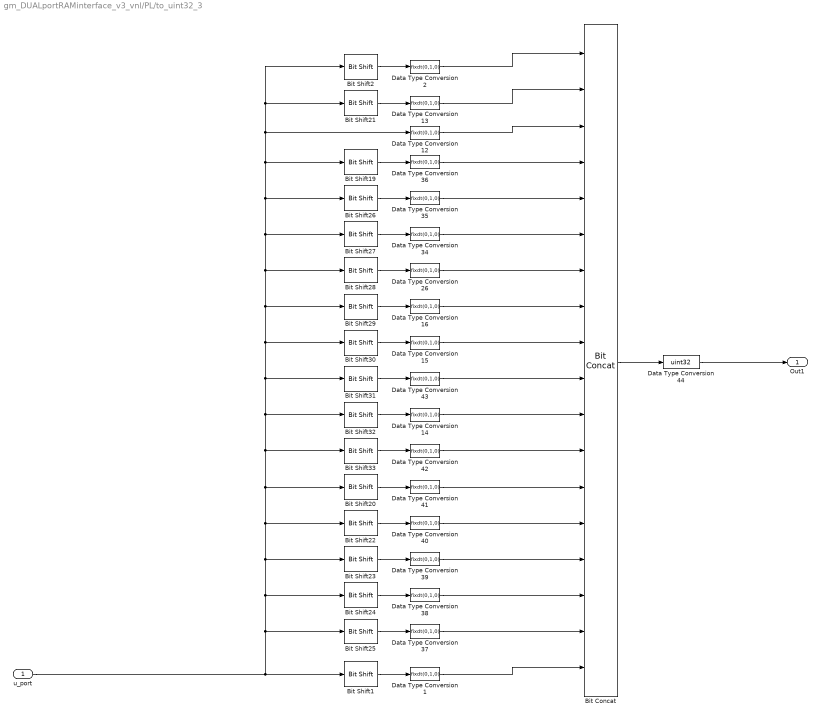
== system gm_DUALportRAMinterface_v3_vnl/PL/to_uint32_3 ==
  u_port : Inport
  Bit Concat : hdlsllib/Logic and Bit Operations/Bit Concat  numInputs=18
  Bit Shift1 : hdlsllib/Logic and Bit Operations/Bit Shift  mode=Shift Left Logical  N=15
  Bit Shift19 : hdlsllib/Logic and Bit Operations/Bit Shift  mode=Shift Left Logical  N=1
  Bit Shift2 : hdlsllib/Logic and Bit Operations/Bit Shift  mode=Shift Right Logical  N=16
  Bit Shift20 : hdlsllib/Logic and Bit Operations/Bit Shift  mode=Shift Left Logical  N=10
  Bit Shift21 : hdlsllib/Logic and Bit Operations/Bit Shift  mode=Shift Right Logical  N=1
  Bit Shift22 : hdlsllib/Logic and Bit Operations/Bit Shift  mode=Shift Left Logical  N=11
  Bit Shift23 : hdlsllib/Logic and Bit Operations/Bit Shift  mode=Shift Left Logical  N=12
  Bit Shift24 : hdlsllib/Logic and Bit Operations/Bit Shift  mode=Shift Left Logical  N=13
  Bit Shift25 : hdlsllib/Logic and Bit Operations/Bit Shift  mode=Shift Left Logical  N=14
  Bit Shift26 : hdlsllib/Logic and Bit Operations/Bit Shift  mode=Shift Left Logical  N=2
  Bit Shift27 : hdlsllib/Logic and Bit Operations/Bit Shift  mode=Shift Left Logical  N=3
  Bit Shift28 : hdlsllib/Logic and Bit Operations/Bit Shift  mode=Shift Left Logical  N=4
  Bit Shift29 : hdlsllib/Logic and Bit Operations/Bit Shift  mode=Shift Left Logical  N=5
  Bit Shift30 : hdlsllib/Logic and Bit Operations/Bit Shift  mode=Shift Left Logical  N=6
  Bit Shift31 : hdlsllib/Logic and Bit Operations/Bit Shift  mode=Shift Left Logical  N=7
  Bit Shift32 : hdlsllib/Logic and Bit Operations/Bit Shift  mode=Shift Left Logical  N=8
  Bit Shift33 : hdlsllib/Logic and Bit Operations/Bit Shift  mode=Shift Left Logical  N=9
  Data Type Conversion{1..2,12..16,26,34..43} (18 alike) : DataTypeConversion  OutDataTypeStr=fixdt(0,1,0)  SaturateOnIntegerOverflow=off  RndMeth=Floor
  Data Type Conversion44 : DataTypeConversion  OutDataTypeStr=uint32  SaturateOnIntegerOverflow=off  RndMeth=Floor
  Out1 : Outport
  wires:
  Bit Concat/1 -> Data Type Conversion44/1
  u_port/1 -> Bit Shift1/1, Bit Shift21/1, Bit Shift2/1, Data Type Conversion12/1, Bit Shift19/1, Bit Shift26/1, Bit Shift27/1, Bit Shift28/1, Bit Shift29/1, Bit Shift30/1, Bit Shift31/1, Bit Shift32/1, Bit Shift33/1, Bit Shift20/1, Bit Shift22/1, Bit Shift23/1, Bit Shift24/1, Bit Shift25/1
  Data Type Conversion14/1 -> Bit Concat/11
  Data Type Conversion1/1 -> Bit Concat/18
  Data Type Conversion2/1 -> Bit Concat/1
  Data Type Conversion26/1 -> Bit Concat/7
  Bit Shift21/1 -> Data Type Conversion13/1
  Data Type Conversion12/1 -> Bit Concat/3
  Bit Shift27/1 -> Data Type Conversion34/1
  Bit Shift22/1 -> Data Type Conversion40/1
  Bit Shift20/1 -> Data Type Conversion41/1
  Bit Shift31/1 -> Data Type Conversion43/1
  Data Type Conversion39/1 -> Bit Concat/15
  Data Type Conversion15/1 -> Bit Concat/9
  Data Type Conversion43/1 -> Bit Concat/10
  Bit Shift33/1 -> Data Type Conversion42/1
  Bit Shift23/1 -> Data Type Conversion39/1
  Bit Shift25/1 -> Data Type Conversion37/1
  Data Type Conversion41/1 -> Bit Concat/13
  Bit Shift2/1 -> Data Type Conversion2/1
  Bit Shift29/1 -> Data Type Conversion16/1
  Bit Shift26/1 -> Data Type Conversion35/1
  Data Type Conversion34/1 -> Bit Concat/6
  Bit Shift28/1 -> Data Type Conversion26/1
  Data Type Conversion36/1 -> Bit Concat/4
  Bit Shift24/1 -> Data Type Conversion38/1
  Bit Shift1/1 -> Data Type Conversion1/1
  Data Type Conversion35/1 -> Bit Concat/5
  Data Type Conversion16/1 -> Bit Concat/8
  Bit Shift19/1 -> Data Type Conversion36/1
  Data Type Conversion13/1 -> Bit Concat/2
  Bit Shift30/1 -> Data Type Conversion15/1
  Data Type Conversion38/1 -> Bit Concat/16
  Data Type Conversion37/1 -> Bit Concat/17
  Data Type Conversion40/1 -> Bit Concat/14
  Bit Shift32/1 -> Data Type Conversion14/1
  Data Type Conversion42/1 -> Bit Concat/12
  Data Type Conversion44/1 -> Out1/1

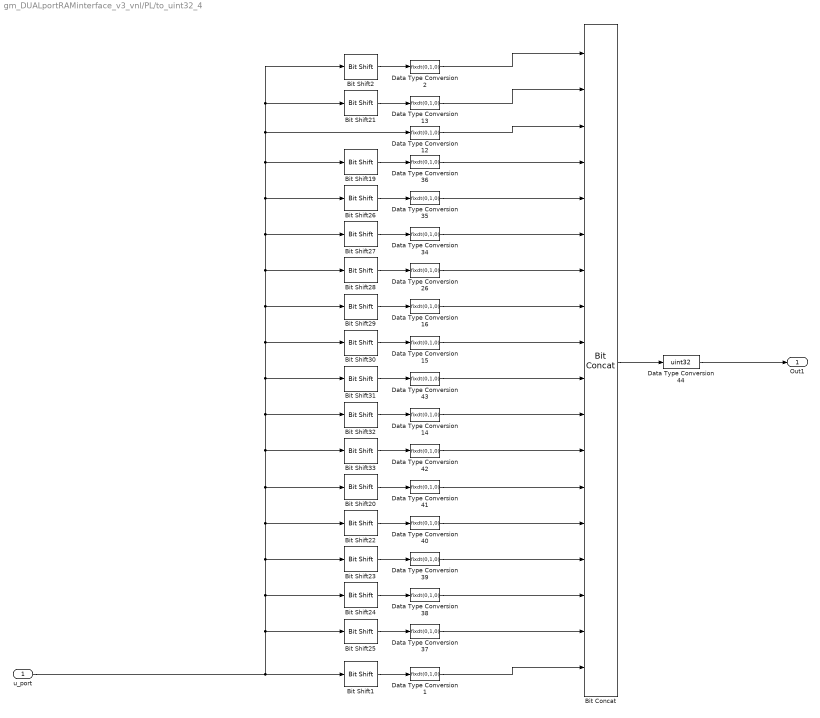
== system gm_DUALportRAMinterface_v3_vnl/PL/to_uint32_4 ==
  u_port : Inport
  Bit Concat : hdlsllib/Logic and Bit Operations/Bit Concat  numInputs=18
  Bit Shift1 : hdlsllib/Logic and Bit Operations/Bit Shift  mode=Shift Left Logical  N=15
  Bit Shift19 : hdlsllib/Logic and Bit Operations/Bit Shift  mode=Shift Left Logical  N=1
  Bit Shift2 : hdlsllib/Logic and Bit Operations/Bit Shift  mode=Shift Right Logical  N=16
  Bit Shift20 : hdlsllib/Logic and Bit Operations/Bit Shift  mode=Shift Left Logical  N=10
  Bit Shift21 : hdlsllib/Logic and Bit Operations/Bit Shift  mode=Shift Right Logical  N=1
  Bit Shift22 : hdlsllib/Logic and Bit Operations/Bit Shift  mode=Shift Left Logical  N=11
  Bit Shift23 : hdlsllib/Logic and Bit Operations/Bit Shift  mode=Shift Left Logical  N=12
  Bit Shift24 : hdlsllib/Logic and Bit Operations/Bit Shift  mode=Shift Left Logical  N=13
  Bit Shift25 : hdlsllib/Logic and Bit Operations/Bit Shift  mode=Shift Left Logical  N=14
  Bit Shift26 : hdlsllib/Logic and Bit Operations/Bit Shift  mode=Shift Left Logical  N=2
  Bit Shift27 : hdlsllib/Logic and Bit Operations/Bit Shift  mode=Shift Left Logical  N=3
  Bit Shift28 : hdlsllib/Logic and Bit Operations/Bit Shift  mode=Shift Left Logical  N=4
  Bit Shift29 : hdlsllib/Logic and Bit Operations/Bit Shift  mode=Shift Left Logical  N=5
  Bit Shift30 : hdlsllib/Logic and Bit Operations/Bit Shift  mode=Shift Left Logical  N=6
  Bit Shift31 : hdlsllib/Logic and Bit Operations/Bit Shift  mode=Shift Left Logical  N=7
  Bit Shift32 : hdlsllib/Logic and Bit Operations/Bit Shift  mode=Shift Left Logical  N=8
  Bit Shift33 : hdlsllib/Logic and Bit Operations/Bit Shift  mode=Shift Left Logical  N=9
  Data Type Conversion{1..2,12..16,26,34..43} (18 alike) : DataTypeConversion  OutDataTypeStr=fixdt(0,1,0)  SaturateOnIntegerOverflow=off  RndMeth=Floor
  Data Type Conversion44 : DataTypeConversion  OutDataTypeStr=uint32  SaturateOnIntegerOverflow=off  RndMeth=Floor
  Out1 : Outport
  wires:
  Data Type Conversion44/1 -> Out1/1
  Data Type Conversion42/1 -> Bit Concat/12
  Bit Shift32/1 -> Data Type Conversion14/1
  Data Type Conversion40/1 -> Bit Concat/14
  Data Type Conversion37/1 -> Bit Concat/17
  Data Type Conversion38/1 -> Bit Concat/16
  Bit Shift30/1 -> Data Type Conversion15/1
  Data Type Conversion13/1 -> Bit Concat/2
  Bit Shift19/1 -> Data Type Conversion36/1
  Data Type Conversion16/1 -> Bit Concat/8
  Data Type Conversion35/1 -> Bit Concat/5
  Bit Shift1/1 -> Data Type Conversion1/1
  Bit Shift24/1 -> Data Type Conversion38/1
  Data Type Conversion36/1 -> Bit Concat/4
  Bit Shift28/1 -> Data Type Conversion26/1
  Data Type Conversion34/1 -> Bit Concat/6
  Bit Shift26/1 -> Data Type Conversion35/1
  Bit Shift29/1 -> Data Type Conversion16/1
  Bit Shift2/1 -> Data Type Conversion2/1
  Data Type Conversion41/1 -> Bit Concat/13
  Bit Shift25/1 -> Data Type Conversion37/1
  Bit Shift23/1 -> Data Type Conversion39/1
  Bit Shift33/1 -> Data Type Conversion42/1
  Data Type Conversion43/1 -> Bit Concat/10
  Data Type Conversion15/1 -> Bit Concat/9
  Data Type Conversion39/1 -> Bit Concat/15
  Bit Shift31/1 -> Data Type Conversion43/1
  Bit Shift20/1 -> Data Type Conversion41/1
  Bit Shift22/1 -> Data Type Conversion40/1
  Bit Shift27/1 -> Data Type Conversion34/1
  Data Type Conversion12/1 -> Bit Concat/3
  Bit Shift21/1 -> Data Type Conversion13/1
  Data Type Conversion26/1 -> Bit Concat/7
  Data Type Conversion2/1 -> Bit Concat/1
  Data Type Conversion1/1 -> Bit Concat/18
  Data Type Conversion14/1 -> Bit Concat/11
  u_port/1 -> Bit Shift25/1, Bit Shift24/1, Bit Shift23/1, Bit Shift22/1, Bit Shift20/1, Bit Shift33/1, Bit Shift32/1, Bit Shift31/1, Bit Shift30/1, Bit Shift29/1, Bit Shift28/1, Bit Shift27/1, Bit Shift26/1, Bit Shift19/1, Data Type Conversion12/1, Bit Shift2/1, Bit Shift21/1, Bit Shift1/1
  Bit Concat/1 -> Data Type Conversion44/1

== system gm_DUALportRAMinterface_v3_vnl/PL/to_uint32_5 ==
  u_port : Inport
  Bit Concat : hdlsllib/Logic and Bit Operations/Bit Concat  numInputs=18
  Bit Shift1 : hdlsllib/Logic and Bit Operations/Bit Shift  mode=Shift Left Logical  N=15
  Bit Shift19 : hdlsllib/Logic and Bit Operations/Bit Shift  mode=Shift Left Logical  N=1
  Bit Shift2 : hdlsllib/Logic and Bit Operations/Bit Shift  mode=Shift Right Logical  N=16
  Bit Shift20 : hdlsllib/Logic and Bit Operations/Bit Shift  mode=Shift Left Logical  N=10
  Bit Shift21 : hdlsllib/Logic and Bit Operations/Bit Shift  mode=Shift Right Logical  N=1
  Bit Shift22 : hdlsllib/Logic and Bit Operations/Bit Shift  mode=Shift Left Logical  N=11
  Bit Shift23 : hdlsllib/Logic and Bit Operations/Bit Shift  mode=Shift Left Logical  N=12
  Bit Shift24 : hdlsllib/Logic and Bit Operations/Bit Shift  mode=Shift Left Logical  N=13
  Bit Shift25 : hdlsllib/Logic and Bit Operations/Bit Shift  mode=Shift Left Logical  N=14
  Bit Shift26 : hdlsllib/Logic and Bit Operations/Bit Shift  mode=Shift Left Logical  N=2
  Bit Shift27 : hdlsllib/Logic and Bit Operations/Bit Shift  mode=Shift Left Logical  N=3
  Bit Shift28 : hdlsllib/Logic and Bit Operations/Bit Shift  mode=Shift Left Logical  N=4
  Bit Shift29 : hdlsllib/Logic and Bit Operations/Bit Shift  mode=Shift Left Logical  N=5
  Bit Shift30 : hdlsllib/Logic and Bit Operations/Bit Shift  mode=Shift Left Logical  N=6
  Bit Shift31 : hdlsllib/Logic and Bit Operations/Bit Shift  mode=Shift Left Logical  N=7
  Bit Shift32 : hdlsllib/Logic and Bit Operations/Bit Shift  mode=Shift Left Logical  N=8
  Bit Shift33 : hdlsllib/Logic and Bit Operations/Bit Shift  mode=Shift Left Logical  N=9
  Data Type Conversion{1..2,12..16,26,34..43} (18 alike) : DataTypeConversion  OutDataTypeStr=fixdt(0,1,0)  SaturateOnIntegerOverflow=off  RndMeth=Floor
  Data Type Conversion44 : DataTypeConversion  OutDataTypeStr=uint32  SaturateOnIntegerOverflow=off  RndMeth=Floor
  Out1 : Outport
  wires:
  Bit Concat/1 -> Data Type Conversion44/1
  u_port/1 -> Bit Shift1/1, Bit Shift21/1, Bit Shift2/1, Data Type Conversion12/1, Bit Shift19/1, Bit Shift26/1, Bit Shift27/1, Bit Shift28/1, Bit Shift29/1, Bit Shift30/1, Bit Shift31/1, Bit Shift32/1, Bit Shift33/1, Bit Shift20/1, Bit Shift22/1, Bit Shift23/1, Bit Shift24/1, Bit Shift25/1
  Data Type Conversion14/1 -> Bit Concat/11
  Data Type Conversion1/1 -> Bit Concat/18
  Data Type Conversion2/1 -> Bit Concat/1
  Data Type Conversion26/1 -> Bit Concat/7
  Bit Shift21/1 -> Data Type Conversion13/1
  Data Type Conversion12/1 -> Bit Concat/3
  Bit Shift27/1 -> Data Type Conversion34/1
  Bit Shift22/1 -> Data Type Conversion40/1
  Bit Shift20/1 -> Data Type Conversion41/1
  Bit Shift31/1 -> Data Type Conversion43/1
  Data Type Conversion39/1 -> Bit Concat/15
  Data Type Conversion15/1 -> Bit Concat/9
  Data Type Conversion43/1 -> Bit Concat/10
  Bit Shift33/1 -> Data Type Conversion42/1
  Bit Shift23/1 -> Data Type Conversion39/1
  Bit Shift25/1 -> Data Type Conversion37/1
  Data Type Conversion41/1 -> Bit Concat/13
  Bit Shift2/1 -> Data Type Conversion2/1
  Bit Shift29/1 -> Data Type Conversion16/1
  Bit Shift26/1 -> Data Type Conversion35/1
  Data Type Conversion34/1 -> Bit Concat/6
  Bit Shift28/1 -> Data Type Conversion26/1
  Data Type Conversion36/1 -> Bit Concat/4
  Bit Shift24/1 -> Data Type Conversion38/1
  Bit Shift1/1 -> Data Type Conversion1/1
  Data Type Conversion35/1 -> Bit Concat/5
  Data Type Conversion16/1 -> Bit Concat/8
  Bit Shift19/1 -> Data Type Conversion36/1
  Data Type Conversion13/1 -> Bit Concat/2
  Bit Shift30/1 -> Data Type Conversion15/1
  Data Type Conversion38/1 -> Bit Concat/16
  Data Type Conversion37/1 -> Bit Concat/17
  Data Type Conversion40/1 -> Bit Concat/14
  Bit Shift32/1 -> Data Type Conversion14/1
  Data Type Conversion42/1 -> Bit Concat/12
  Data Type Conversion44/1 -> Out1/1

== system gm_DUALportRAMinterface_v3_vnl/PL/to_uint32_6 ==
  u_port : Inport
  Bit Concat : hdlsllib/Logic and Bit Operations/Bit Concat  numInputs=18
  Bit Shift1 : hdlsllib/Logic and Bit Operations/Bit Shift  mode=Shift Left Logical  N=15
  Bit Shift19 : hdlsllib/Logic and Bit Operations/Bit Shift  mode=Shift Left Logical  N=1
  Bit Shift2 : hdlsllib/Logic and Bit Operations/Bit Shift  mode=Shift Right Logical  N=16
  Bit Shift20 : hdlsllib/Logic and Bit Operations/Bit Shift  mode=Shift Left Logical  N=10
  Bit Shift21 : hdlsllib/Logic and Bit Operations/Bit Shift  mode=Shift Right Logical  N=1
  Bit Shift22 : hdlsllib/Logic and Bit Operations/Bit Shift  mode=Shift Left Logical  N=11
  Bit Shift23 : hdlsllib/Logic and Bit Operations/Bit Shift  mode=Shift Left Logical  N=12
  Bit Shift24 : hdlsllib/Logic and Bit Operations/Bit Shift  mode=Shift Left Logical  N=13
  Bit Shift25 : hdlsllib/Logic and Bit Operations/Bit Shift  mode=Shift Left Logical  N=14
  Bit Shift26 : hdlsllib/Logic and Bit Operations/Bit Shift  mode=Shift Left Logical  N=2
  Bit Shift27 : hdlsllib/Logic and Bit Operations/Bit Shift  mode=Shift Left Logical  N=3
  Bit Shift28 : hdlsllib/Logic and Bit Operations/Bit Shift  mode=Shift Left Logical  N=4
  Bit Shift29 : hdlsllib/Logic and Bit Operations/Bit Shift  mode=Shift Left Logical  N=5
  Bit Shift30 : hdlsllib/Logic and Bit Operations/Bit Shift  mode=Shift Left Logical  N=6
  Bit Shift31 : hdlsllib/Logic and Bit Operations/Bit Shift  mode=Shift Left Logical  N=7
  Bit Shift32 : hdlsllib/Logic and Bit Operations/Bit Shift  mode=Shift Left Logical  N=8
  Bit Shift33 : hdlsllib/Logic and Bit Operations/Bit Shift  mode=Shift Left Logical  N=9
  Data Type Conversion{1..2,12..16,26,34..43} (18 alike) : DataTypeConversion  OutDataTypeStr=fixdt(0,1,0)  SaturateOnIntegerOverflow=off  RndMeth=Floor
  Data Type Conversion44 : DataTypeConversion  OutDataTypeStr=uint32  SaturateOnIntegerOverflow=off  RndMeth=Floor
  Out1 : Outport
  wires:
  Data Type Conversion44/1 -> Out1/1
  Data Type Conversion42/1 -> Bit Concat/12
  Bit Shift32/1 -> Data Type Conversion14/1
  Data Type Conversion40/1 -> Bit Concat/14
  Data Type Conversion37/1 -> Bit Concat/17
  Data Type Conversion38/1 -> Bit Concat/16
  Bit Shift30/1 -> Data Type Conversion15/1
  Data Type Conversion13/1 -> Bit Concat/2
  Bit Shift19/1 -> Data Type Conversion36/1
  Data Type Conversion16/1 -> Bit Concat/8
  Data Type Conversion35/1 -> Bit Concat/5
  Bit Shift1/1 -> Data Type Conversion1/1
  Bit Shift24/1 -> Data Type Conversion38/1
  Data Type Conversion36/1 -> Bit Concat/4
  Bit Shift28/1 -> Data Type Conversion26/1
  Data Type Conversion34/1 -> Bit Concat/6
  Bit Shift26/1 -> Data Type Conversion35/1
  Bit Shift29/1 -> Data Type Conversion16/1
  Bit Shift2/1 -> Data Type Conversion2/1
  Data Type Conversion41/1 -> Bit Concat/13
  Bit Shift25/1 -> Data Type Conversion37/1
  Bit Shift23/1 -> Data Type Conversion39/1
  Bit Shift33/1 -> Data Type Conversion42/1
  Data Type Conversion43/1 -> Bit Concat/10
  Data Type Conversion15/1 -> Bit Concat/9
  Data Type Conversion39/1 -> Bit Concat/15
  Bit Shift31/1 -> Data Type Conversion43/1
  Bit Shift20/1 -> Data Type Conversion41/1
  Bit Shift22/1 -> Data Type Conversion40/1
  Bit Shift27/1 -> Data Type Conversion34/1
  Data Type Conversion12/1 -> Bit Concat/3
  Bit Shift21/1 -> Data Type Conversion13/1
  Data Type Conversion26/1 -> Bit Concat/7
  Data Type Conversion2/1 -> Bit Concat/1
  Data Type Conversion1/1 -> Bit Concat/18
  Data Type Conversion14/1 -> Bit Concat/11
  u_port/1 -> Bit Shift25/1, Bit Shift24/1, Bit Shift23/1, Bit Shift22/1, Bit Shift20/1, Bit Shift33/1, Bit Shift32/1, Bit Shift31/1, Bit Shift30/1, Bit Shift29/1, Bit Shift28/1, Bit Shift27/1, Bit Shift26/1, Bit Shift19/1, Data Type Conversion12/1, Bit Shift2/1, Bit Shift21/1, Bit Shift1/1
  Bit Concat/1 -> Data Type Conversion44/1

== system gm_DUALportRAMinterface_v3_vnl/PL/Compare/Assert_Out1 ==
  cosim : Inport
  dut : Inport  Port=2
  AssertEq : Assertion  StopWhenAssertionFail=off
  Compare To Zero : simulink/Logic and Bit Operations/Compare To Zero  relop===  OutDataTypeStr=boolean
  Relational Operator : RelationalOperator  Operator===  OutDataTypeStr=boolean  InputSameDT=off
  compare: Out1 : Scope  NumInputPorts=3
  wires:
  Compare To Zero/1 -> compare: Out1/3  "err"
  Relational Operator/1 -> Compare To Zero/1, AssertEq/1
  cosim/1 -> compare: Out1/1, Relational Operator/1  "cosim"
  dut/1 -> compare: Out1/2, Relational Operator/2  "dut ref"

== system gm_DUALportRAMinterface_v3_vnl/PL/Compare/CleanupScopes ==

== system gm_DUALportRAMinterface_v3_vnl/PL/Compare/Enable ==
